simulink model "Flexible_Beam_LP_Modes_GenSS"  (R2017a)
settings: Solver=ode23t  StartTime=0.0  StopTime=200  RelTol=1e-3  AbsTol=1e-6  EnableMultiTasking=on
PreLoadFcn:
  | flexBeam_default_parameters
PostLoadFcn:
  | warning off Simulink:Engine:UsingDefaultMaxStepSize
  | warning off Simulink:Engine:SaveWithParameterizedLinks_Warning
undefined symbols (not defined in the file): beam_length, beam_wall, beam_width, Damping, density, Extr_Data_Box, extrusion_data_def, kbendingx, kbendingy, kelongz, ktwistz, num_elem, shearM, X, Y, youngsM, Z
libraries: sm_lib x307, nesl_utility x65
(part 1 of 9)
CloseFcn:
  | try,close(h1_Flexible_Beam_LP),end
  | clear h1_Flexible_Beam_LP
Description:
  | Lumped Parameter Beam for State Space Calculation
  | 
  | Copyright 2014-2017 The MathWorks, Inc.
settings Model: Creator=smiller  LastModifiedBy=smiller
settings DataIOCC: LimitDataPoints=on  SaveFormat=Array
settings OptimizationCC: LifeSpan=inf
settings DebuggingCC: UnderspecifiedInitializationDetection=Classic  MergeDetectMultiDrivingBlocksExec=none  SolverPrmCheckMsg=warning  AllowSymbolicDim=off  StateNameClashWarn=warning  SFUnexpectedBacktrackingDiag=warning  SFNoUnconditionalDefaultTransitionDiag=warning  SFExecutionAtInitializationDiag=none
settings HardwareCC: ProdBitPerPointer=32  ProdBitPerSizeT=32  ProdBitPerPtrDiffT=32  ProdLargestAtomicFloat=None  ProdIntDivRoundTo=Undefined  ProdEndianess=Unspecified  ProdWordSize=32  ProdHWDeviceType=32-bit Generic
settings ModelReferenceCC: PropagateSignalLabelsOutOfModel=off
settings GRTTargetCC: TargetLangStandard=C89/C90 (ANSI)  GeneratePreprocessorConditionals=Disable all
settings ConfigComp: CovMetricSettings=dw  CovHtmlReporting=on  CovSaveCumulativeToWorkspaceVar=on  CovSaveSingleToWorkspaceVar=on  CovExternalEMLEnable=off  CovSFcnEnable=off
settings ConfigurationSet: Description=SimMechanics 2G
settings ExplorerConfigSet: InternalSimMechanicsExplorerSettings="<ExplorerConfiguration><canonicalview>default</canonicalview><AnimationSetting><BasePlaybackSpeed>1.0</BasePlaybackSpeed><PlaybackSpeedFactor>1.0</PlaybackSpeedFactor></AnimationSetting><TilePanel><TileInfo><Tiles Columns=\"1\" Count=\"1\" Rows=\"1\"><Column Left=\"2\" Weight=\"1\"/><Column Left=\"626\"/><Row Top=\"2\" Weight=\"1\"/><Row Top=\"393\"/><Tile Height=\"1\" Width=\"1\" X=\"0\" Y=\"0\"/></Tiles></TileInfo><SceneInfo><SceneViewer><BGColor><R>0.60000002384185791</R><G>0.60000002384185791</G><B>0.60000002384185791</B></BGColor><Camera><Position><X>46.619711055341185</X><Y>-0.34983005837123721</Y><Z>0.38649668367083467</Z></Position><Center><X>15.061424751729401</X><Y>-0.47805428343950285</Y><Z>0.22325866927449958</Z></Center><Up><X>-0.0040752125209600008</X><Y>0.99998893056788307</Y><Z>0.0023518895830039648</Z></Up><Left>-1.9626362085342408</Left><Right>1.9626362085342408</Right><Bottom>-0.98671855330467229</Bottom><Top>0.98671855330467229</Top></Camera></SceneViewer></SceneInfo></TilePanel></ExplorerConfiguration>"

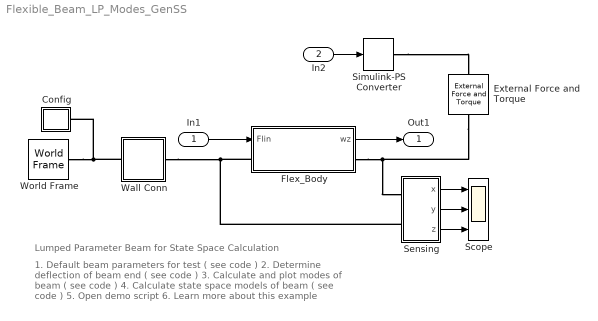
== system Flexible_Beam_LP_Modes_GenSS ==
  note: Lumped Parameter Beam for State Space Calculation
  note: 1. Default beam parameters for test ( see code )
      | 2. Determine deflection of beam end ( see code )
      | 3. Calculate and plot modes of beam ( see code )
      | 4. Calculate state space models of beam ( see code )
      | 5. Open demo script
      | 6. Learn more about this example
  In1 : Inport
  In2 : Inport  Port=2
  Config : Subsystem
  External Force and Torque : sm_lib/Forces and Torques/External Force and Torque  ForceResolutionFrame=AttachedFrame  EnableForceX=off  EnableForceY=on  EnableForceZ=off  EnableForce=off  TorqueResolutionFrame=AttachedFrame  EnableTorqueX=off  EnableTorqueY=off  EnableTorqueZ=off  EnableTorque=off
  Flex_Body : Subsystem  mask(Flexible Body){rho=density, youngsM=youngsM, shearM=shearM, b=Damping, popup_xc=Hollow Rectangle, beam_width=beam_width, beam_width_in=beam_width-2*beam_wall, beam_height=beam_width, beam_height_in=beam_width-2*beam_wall, circle_diameter=beam_width, circle_diameter_in=beam_width-2*beam_wall, custom_ixx=2.6121e-003, custom_iyy=2.6121e-003, custom_j=5.2242e-003, extrusion_data_custom=extrusion_data_def, beam_length=beam_length, numelem=num_elem, extrusion_data=Extr_Data_Box(beam_width,beam_width-2*beam_wall,beam_width,beam_width-2*beam_wall), radio_flextype=3-Axis Bending, Elongation, checkbox_lin=on}
      mask prompts: rho "Material Density (kg/(m^3)"; youngsM "Modulus of Elasticity (N/m2)"; shearM "Shear Modulus (N/m2)"; b "Damping Constant (Nm/rad.s)"; popup_xc "Cross-Section Type"; custom_ixx "Area Ixx"; custom_iyy "Area Iyy"; custom_j "Polar J"; extrusion_data_custom "Extrusion data [x;y] (m)"; beam_length "Length (m)"; numelem "Number of elements"; radio_flextype "Flexibility Type"; checkbox_lin "Add connections for linearization"
      mask help: Models a flexible beam based on lumped parameter method. Number of flexible elements, material properties as well as beam cross section and dimensions can be varied from mask parameters.
      mask init:
      | if(popup_xc==1)
      |     extrusion_data = Extr_Data_Box(beam_width,beam_width_in,beam_height,beam_height_in);
      |     xc_props = [beam_width beam_width_in beam_height beam_height_in];
      | elseif(popup_xc==2)
      |     extrusion_data = Extr_Data_Ring(circle_diameter/2,circle_diameter_in/2,0,360);
      |     xc_props = [circle_diameter circle_diameter_in];
      | elseif(popup_xc==3)
      |     extrusion_data = extrusion_data_custom;
      |     extrusion_data_vec = reshape(extrusion_data,[length(extrusion_data)*2,1]);
      |     xc_props = [custom_ixx;custom_iyy;custom_j;extrusion_data_vec];
      | end
      | 
      | [kbendingx, kbendingy, ktwistz, kelongz, length] = ...
      |     Compute_GFE_Prop(youngsM, shearM, numelem, beam_length,popup_xc,...
      |     xc_props);
      | 
      | flexBeam_lpar_construct_beam(gcb,numelem,radio_flextype,checkbox_lin);
      | 
      | state_order = flexBeam_lpar_getstateorder(gcb);
      | assignin('base','state_order',state_order);
      | 
      | clear xc_props
      settings: AttributesFormatString=No of Elem: 30  CopyFcn=set_param(gcb, 'LinkStatus', 'none')
      mask TypeOptions popup_xc: Hollow Rectangle | Hollow Circle | Custom
      mask Callback popup_xc:
      | maskObj = Simulink.Mask.get(gcb);
      | rcti_h = maskObj.getDialogControl('container_rectimage');
      | rctp_h = maskObj.getDialogControl('container_rectparams');
      | ciri_h = maskObj.getDialogControl('container_circleimage');
      | cirp_h = maskObj.getDialogControl('container_circleparams');
      | cusi_h = maskObj.getDialogControl('container_customimage');
      | cusp_h = maskObj.getDialogControl('container_customparams');
      | 
      | rcti_h.Visible = 'off';
      | rctp_h.Visible = 'off';
      | ciri_h.Visible = 'off';
      | cirp_h.Visible = 'off';
      | cusi_h.Visible = 'off';
      | cusp_h.Visible = 'off';
      | 
      | if strcmp(get_param(gcb,'popup_xc'),'Hollow Rectangle')
      |     rcti_h.Visible = 'on';
      |     rctp_h.Visible = 'on';
      | elseif strcmp(get_param(gcb,'popup_xc'),'Hollow Circle')
      |     ciri_h.Visible = 'on';
      |     cirp_h.Visible = 'on';
      | elseif strcmp(get_param(gcb,'popup_xc'),'Custom')
      |     cusi_h.Visible = 'on';
      |     cusp_h.Visible = 'on';
      | end
      | 
      | clear rcti_h rctp_h ciri_h cirp_h cusi_h cusp_h
      mask TypeOptions radio_flextype: 1-Axis Bending | 3-Axis Bending, Elongation
      mask DialogControl text_outer Prompt: Outer
      mask DialogControl text_inner Prompt: Inner
      mask DialogControl text_width Prompt: Width (m)
      mask DialogControl text_height Prompt: Height (m)
      mask DialogControl text_circle_outer Prompt: Outer
      mask DialogControl text_circle_inner Prompt: Inner
      mask DialogControl text_circle_width Prompt: Diameter (m)
      mask DialogControl text_moi Prompt: Moment of Inertia (m^4)
      mask DialogControl push_configBeam Prompt: Configure Beam
      mask DialogControl push_configBeam Callback:
      | thisblock = gcb;
      | v = get_param(thisblock,'MaskWSVariables');
      | getMaskValue = containers.Map({v.Name}',{v.Value}');
      | nelem = getMaskValue('numelem');
      | ftype = getMaskValue('radio_flextype');
      | flexBeam_lpar_construct_beam(thisblock,nelem,ftype,1)
      | %{
      | flexBeam_lpar_assemble_elements_4lin(thisblock,nelem);
      | ftype = getMaskValue('radio_flextype');
      | flexBeam_lpar_configure_flextype(thisblock,ftype);
      | %}
      | clear maskObj nel_h ftype thisblock
      mask Display: image(imread('Flexible_Beam.png'));
  Scope : Scope  NumInputPorts=3
  Sensing : Subsystem
  Simulink-PS Converter : nesl_utility/Simulink-PS Converter  PhysicalDomain=network_engine_domain  SubClassName=ps_input  LeftPortType=input  RightPortType=output  PseudoPeriodic=off  Frequencies=[]  NoiseDistribution=none  NoiseParameters=[]  Unit=1  AffineConversion=off  FilteringAndDerivatives=zero  SimscapeFilterOrder=1  InputFilterTimeConstant=0.001  UdotUserProvided=1
  Wall Conn : Subsystem  Variant=on  OverrideUsingVariant=Rotate
      mask Display:
      | blk = find_system(gcbh, 'SearchDepth', 1, 'Parent', gcb, 'VariantObject', get_param(gcb,'activevariant'));
      | eval(get_param(blk, 'MaskDisplay'));
  World Frame : sm_lib/Frames and Transforms/World Frame
  Out1 : Outport
  wires:
  In2/1 -> Simulink-PS Converter/1
  Sensing/1(x) -> Scope/1
  Sensing/2(y) -> Scope/2
  Sensing/3(z) -> Scope/3
  In1/1 -> Flex_Body/1(Flin)
  Flex_Body/1(wz) -> Out1/1
  connections:
  Simulink-PS Converter/RConn1 -- External Force and Torque/LConn1
  External Force and Torque/RConn1 -- Flex_Body/RConn1 -- Sensing/LConn1
  Sensing/LConn2 -- Flex_Body/LConn1 -- Wall Conn/RConn1
  World Frame/RConn1 -- Config/LConn1 -- Wall Conn/LConn1

== system Flexible_Beam_LP_Modes_GenSS/Config ==
  Mechanism Configuration : sm_lib/Utilities/Mechanism Configuration  UniformGravity=Constant  GravityVector=gravity  GravityUnits=m/s^2  LinearizationDelta=0.001
  Solver Configuration : nesl_utility/Solver Configuration  PhysicalDomain=network_engine_domain  SubClassName=solver  LeftPortType=input  RightPortType=generic  Accelerate=off  Tones=[]  Harmonics=[]  SimulateNoise=off  Profile=off  UseLocalSampling=off  EnableSwitchedLinearOptims=on  FrequencyDomain=off  UseCCode=off  RelTol=0.001  AbsTol=1e-06  MinStep=1e-09  ToWorkspace=off  RevertToSquareIcSolve=off  NumHomotopyIterations=100  PhasorMode=off  PhasorModeNumHarmonics=1  OverrideAbsTol=off  DoDC=off  ResidualTolerance=1e-09  UseLocalSolver=off  LocalSolverChoice=NE_BACKWARD_EULER_ADVANCER  LocalSolverSampleTime=0.001  DoFixedCost=off  MaxNonlinIter=3  MaxModeIter=2  LinearAlgebra=Sparse  DelaysMemoryBudget=1024  AutomaticFiltering=on  FilteringTimeConstant=0.001
  C : PMIOPort  Port=1  Side=Left
  connections:
  Mechanism Configuration/RConn1 -- Solver Configuration/RConn1 -- C/RConn1

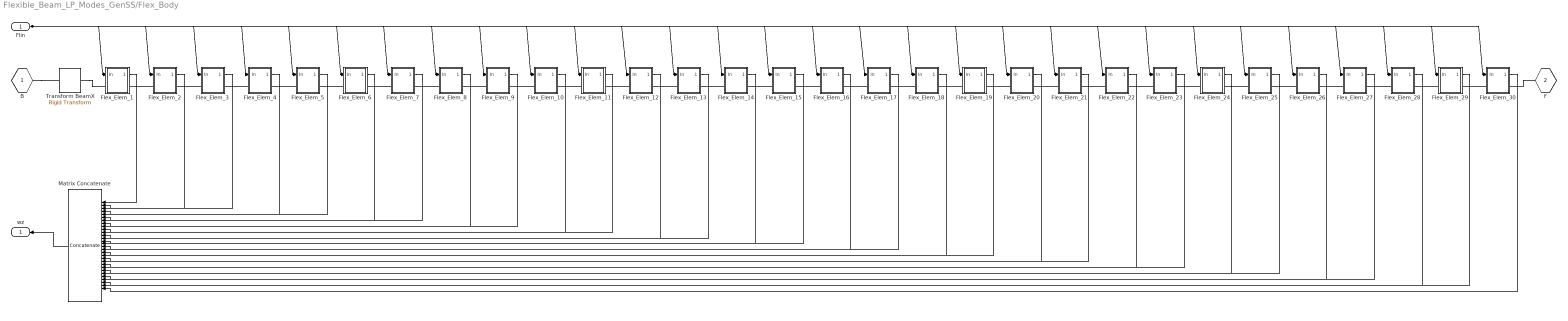
== system Flexible_Beam_LP_Modes_GenSS/Flex_Body ==
  Flin : Inport
  Flex_Elem_1 : Subsystem  VariantControl=Bend  mask{length=length, rho=rho, beam_width=beam_width, beam_wall=beam_wall, kbendingx=kbendingx, kbendingy=kbendingy, kbendingz=ktwistz, kelongz=kelongz, b=b}
      mask prompts: length "Beam Length (m)"; rho "Material Density (kg/(m^3)"; beam_width "Beam Width & Height (m)"; beam_wall "Beam Wall Thickness (m)"; kbendingx "Bending Spring Constant about X(Nm/rad)"; kbendingy "Bending Spring Constant about Y(Nm/rad)"; kbendingz "Twist Spring Constant about Z(Nm/rad)"; kelongz "Elongation Spring Constant about Z(N/m)"; b "Damping Constant (Nm/rad.s)"
      settings: CopyFcn=set_param(gcb, 'LinkStatus', 'none')
  Flex_Elem_10 : Subsystem  VariantControl=Bend  mask{length=length, rho=rho, beam_width=beam_width, beam_wall=beam_wall, kbendingx=kbendingx, kbendingy=kbendingy, kbendingz=ktwistz, kelongz=kelongz, b=b}
      mask prompts: length "Beam Length (m)"; rho "Material Density (kg/(m^3)"; beam_width "Beam Width & Height (m)"; beam_wall "Beam Wall Thickness (m)"; kbendingx "Bending Spring Constant about X(Nm/rad)"; kbendingy "Bending Spring Constant about Y(Nm/rad)"; kbendingz "Twist Spring Constant about Z(Nm/rad)"; kelongz "Elongation Spring Constant about Z(N/m)"; b "Damping Constant (Nm/rad.s)"
      settings: CopyFcn=set_param(gcb, 'LinkStatus', 'none')
  Flex_Elem_11 : Subsystem  VariantControl=Bend  mask{length=length, rho=rho, beam_width=beam_width, beam_wall=beam_wall, kbendingx=kbendingx, kbendingy=kbendingy, kbendingz=ktwistz, kelongz=kelongz, b=b}
      mask prompts: length "Beam Length (m)"; rho "Material Density (kg/(m^3)"; beam_width "Beam Width & Height (m)"; beam_wall "Beam Wall Thickness (m)"; kbendingx "Bending Spring Constant about X(Nm/rad)"; kbendingy "Bending Spring Constant about Y(Nm/rad)"; kbendingz "Twist Spring Constant about Z(Nm/rad)"; kelongz "Elongation Spring Constant about Z(N/m)"; b "Damping Constant (Nm/rad.s)"
      settings: CopyFcn=set_param(gcb, 'LinkStatus', 'none')
  Flex_Elem_12 : Subsystem  VariantControl=Bend  mask{length=length, rho=rho, beam_width=beam_width, beam_wall=beam_wall, kbendingx=kbendingx, kbendingy=kbendingy, kbendingz=ktwistz, kelongz=kelongz, b=b}
      mask prompts: length "Beam Length (m)"; rho "Material Density (kg/(m^3)"; beam_width "Beam Width & Height (m)"; beam_wall "Beam Wall Thickness (m)"; kbendingx "Bending Spring Constant about X(Nm/rad)"; kbendingy "Bending Spring Constant about Y(Nm/rad)"; kbendingz "Twist Spring Constant about Z(Nm/rad)"; kelongz "Elongation Spring Constant about Z(N/m)"; b "Damping Constant (Nm/rad.s)"
      settings: CopyFcn=set_param(gcb, 'LinkStatus', 'none')
  Flex_Elem_13 : Subsystem  VariantControl=Bend  mask{length=length, rho=rho, beam_width=beam_width, beam_wall=beam_wall, kbendingx=kbendingx, kbendingy=kbendingy, kbendingz=ktwistz, kelongz=kelongz, b=b}
      mask prompts: length "Beam Length (m)"; rho "Material Density (kg/(m^3)"; beam_width "Beam Width & Height (m)"; beam_wall "Beam Wall Thickness (m)"; kbendingx "Bending Spring Constant about X(Nm/rad)"; kbendingy "Bending Spring Constant about Y(Nm/rad)"; kbendingz "Twist Spring Constant about Z(Nm/rad)"; kelongz "Elongation Spring Constant about Z(N/m)"; b "Damping Constant (Nm/rad.s)"
      settings: CopyFcn=set_param(gcb, 'LinkStatus', 'none')
  Flex_Elem_14 : Subsystem  VariantControl=Bend  mask{length=length, rho=rho, beam_width=beam_width, beam_wall=beam_wall, kbendingx=kbendingx, kbendingy=kbendingy, kbendingz=ktwistz, kelongz=kelongz, b=b}
      mask prompts: length "Beam Length (m)"; rho "Material Density (kg/(m^3)"; beam_width "Beam Width & Height (m)"; beam_wall "Beam Wall Thickness (m)"; kbendingx "Bending Spring Constant about X(Nm/rad)"; kbendingy "Bending Spring Constant about Y(Nm/rad)"; kbendingz "Twist Spring Constant about Z(Nm/rad)"; kelongz "Elongation Spring Constant about Z(N/m)"; b "Damping Constant (Nm/rad.s)"
      settings: CopyFcn=set_param(gcb, 'LinkStatus', 'none')
  Flex_Elem_15 : Subsystem  VariantControl=Bend  mask{length=length, rho=rho, beam_width=beam_width, beam_wall=beam_wall, kbendingx=kbendingx, kbendingy=kbendingy, kbendingz=ktwistz, kelongz=kelongz, b=b}
      mask prompts: length "Beam Length (m)"; rho "Material Density (kg/(m^3)"; beam_width "Beam Width & Height (m)"; beam_wall "Beam Wall Thickness (m)"; kbendingx "Bending Spring Constant about X(Nm/rad)"; kbendingy "Bending Spring Constant about Y(Nm/rad)"; kbendingz "Twist Spring Constant about Z(Nm/rad)"; kelongz "Elongation Spring Constant about Z(N/m)"; b "Damping Constant (Nm/rad.s)"
      settings: CopyFcn=set_param(gcb, 'LinkStatus', 'none')
  Flex_Elem_16 : Subsystem  VariantControl=Bend  mask{length=length, rho=rho, beam_width=beam_width, beam_wall=beam_wall, kbendingx=kbendingx, kbendingy=kbendingy, kbendingz=ktwistz, kelongz=kelongz, b=b}
      mask prompts: length "Beam Length (m)"; rho "Material Density (kg/(m^3)"; beam_width "Beam Width & Height (m)"; beam_wall "Beam Wall Thickness (m)"; kbendingx "Bending Spring Constant about X(Nm/rad)"; kbendingy "Bending Spring Constant about Y(Nm/rad)"; kbendingz "Twist Spring Constant about Z(Nm/rad)"; kelongz "Elongation Spring Constant about Z(N/m)"; b "Damping Constant (Nm/rad.s)"
      settings: CopyFcn=set_param(gcb, 'LinkStatus', 'none')
  Flex_Elem_17 : Subsystem  VariantControl=Bend  mask{length=length, rho=rho, beam_width=beam_width, beam_wall=beam_wall, kbendingx=kbendingx, kbendingy=kbendingy, kbendingz=ktwistz, kelongz=kelongz, b=b}
      mask prompts: length "Beam Length (m)"; rho "Material Density (kg/(m^3)"; beam_width "Beam Width & Height (m)"; beam_wall "Beam Wall Thickness (m)"; kbendingx "Bending Spring Constant about X(Nm/rad)"; kbendingy "Bending Spring Constant about Y(Nm/rad)"; kbendingz "Twist Spring Constant about Z(Nm/rad)"; kelongz "Elongation Spring Constant about Z(N/m)"; b "Damping Constant (Nm/rad.s)"
      settings: CopyFcn=set_param(gcb, 'LinkStatus', 'none')
  Flex_Elem_18 : Subsystem  VariantControl=Bend  mask{length=length, rho=rho, beam_width=beam_width, beam_wall=beam_wall, kbendingx=kbendingx, kbendingy=kbendingy, kbendingz=ktwistz, kelongz=kelongz, b=b}
      mask prompts: length "Beam Length (m)"; rho "Material Density (kg/(m^3)"; beam_width "Beam Width & Height (m)"; beam_wall "Beam Wall Thickness (m)"; kbendingx "Bending Spring Constant about X(Nm/rad)"; kbendingy "Bending Spring Constant about Y(Nm/rad)"; kbendingz "Twist Spring Constant about Z(Nm/rad)"; kelongz "Elongation Spring Constant about Z(N/m)"; b "Damping Constant (Nm/rad.s)"
      settings: CopyFcn=set_param(gcb, 'LinkStatus', 'none')
  Flex_Elem_19 : Subsystem  VariantControl=Bend  mask{length=length, rho=rho, beam_width=beam_width, beam_wall=beam_wall, kbendingx=kbendingx, kbendingy=kbendingy, kbendingz=ktwistz, kelongz=kelongz, b=b}
      mask prompts: length "Beam Length (m)"; rho "Material Density (kg/(m^3)"; beam_width "Beam Width & Height (m)"; beam_wall "Beam Wall Thickness (m)"; kbendingx "Bending Spring Constant about X(Nm/rad)"; kbendingy "Bending Spring Constant about Y(Nm/rad)"; kbendingz "Twist Spring Constant about Z(Nm/rad)"; kelongz "Elongation Spring Constant about Z(N/m)"; b "Damping Constant (Nm/rad.s)"
      settings: CopyFcn=set_param(gcb, 'LinkStatus', 'none')
  Flex_Elem_2 : Subsystem  VariantControl=Bend  mask{length=length, rho=rho, beam_width=beam_width, beam_wall=beam_wall, kbendingx=kbendingx, kbendingy=kbendingy, kbendingz=ktwistz, kelongz=kelongz, b=b}
      mask prompts: length "Beam Length (m)"; rho "Material Density (kg/(m^3)"; beam_width "Beam Width & Height (m)"; beam_wall "Beam Wall Thickness (m)"; kbendingx "Bending Spring Constant about X(Nm/rad)"; kbendingy "Bending Spring Constant about Y(Nm/rad)"; kbendingz "Twist Spring Constant about Z(Nm/rad)"; kelongz "Elongation Spring Constant about Z(N/m)"; b "Damping Constant (Nm/rad.s)"
      settings: CopyFcn=set_param(gcb, 'LinkStatus', 'none')
  Flex_Elem_20 : Subsystem  VariantControl=Bend  mask{length=length, rho=rho, beam_width=beam_width, beam_wall=beam_wall, kbendingx=kbendingx, kbendingy=kbendingy, kbendingz=ktwistz, kelongz=kelongz, b=b}
      mask prompts: length "Beam Length (m)"; rho "Material Density (kg/(m^3)"; beam_width "Beam Width & Height (m)"; beam_wall "Beam Wall Thickness (m)"; kbendingx "Bending Spring Constant about X(Nm/rad)"; kbendingy "Bending Spring Constant about Y(Nm/rad)"; kbendingz "Twist Spring Constant about Z(Nm/rad)"; kelongz "Elongation Spring Constant about Z(N/m)"; b "Damping Constant (Nm/rad.s)"
      settings: CopyFcn=set_param(gcb, 'LinkStatus', 'none')
  Flex_Elem_21 : Subsystem  VariantControl=Bend  mask{length=length, rho=rho, beam_width=beam_width, beam_wall=beam_wall, kbendingx=kbendingx, kbendingy=kbendingy, kbendingz=ktwistz, kelongz=kelongz, b=b}
      mask prompts: length "Beam Length (m)"; rho "Material Density (kg/(m^3)"; beam_width "Beam Width & Height (m)"; beam_wall "Beam Wall Thickness (m)"; kbendingx "Bending Spring Constant about X(Nm/rad)"; kbendingy "Bending Spring Constant about Y(Nm/rad)"; kbendingz "Twist Spring Constant about Z(Nm/rad)"; kelongz "Elongation Spring Constant about Z(N/m)"; b "Damping Constant (Nm/rad.s)"
      settings: CopyFcn=set_param(gcb, 'LinkStatus', 'none')
  Flex_Elem_22 : Subsystem  VariantControl=Bend  mask{length=length, rho=rho, beam_width=beam_width, beam_wall=beam_wall, kbendingx=kbendingx, kbendingy=kbendingy, kbendingz=ktwistz, kelongz=kelongz, b=b}
      mask prompts: length "Beam Length (m)"; rho "Material Density (kg/(m^3)"; beam_width "Beam Width & Height (m)"; beam_wall "Beam Wall Thickness (m)"; kbendingx "Bending Spring Constant about X(Nm/rad)"; kbendingy "Bending Spring Constant about Y(Nm/rad)"; kbendingz "Twist Spring Constant about Z(Nm/rad)"; kelongz "Elongation Spring Constant about Z(N/m)"; b "Damping Constant (Nm/rad.s)"
      settings: CopyFcn=set_param(gcb, 'LinkStatus', 'none')
  Flex_Elem_23 : Subsystem  VariantControl=Bend  mask{length=length, rho=rho, beam_width=beam_width, beam_wall=beam_wall, kbendingx=kbendingx, kbendingy=kbendingy, kbendingz=ktwistz, kelongz=kelongz, b=b}
      mask prompts: length "Beam Length (m)"; rho "Material Density (kg/(m^3)"; beam_width "Beam Width & Height (m)"; beam_wall "Beam Wall Thickness (m)"; kbendingx "Bending Spring Constant about X(Nm/rad)"; kbendingy "Bending Spring Constant about Y(Nm/rad)"; kbendingz "Twist Spring Constant about Z(Nm/rad)"; kelongz "Elongation Spring Constant about Z(N/m)"; b "Damping Constant (Nm/rad.s)"
      settings: CopyFcn=set_param(gcb, 'LinkStatus', 'none')
  Flex_Elem_24 : Subsystem  VariantControl=Bend  mask{length=length, rho=rho, beam_width=beam_width, beam_wall=beam_wall, kbendingx=kbendingx, kbendingy=kbendingy, kbendingz=ktwistz, kelongz=kelongz, b=b}
      mask prompts: length "Beam Length (m)"; rho "Material Density (kg/(m^3)"; beam_width "Beam Width & Height (m)"; beam_wall "Beam Wall Thickness (m)"; kbendingx "Bending Spring Constant about X(Nm/rad)"; kbendingy "Bending Spring Constant about Y(Nm/rad)"; kbendingz "Twist Spring Constant about Z(Nm/rad)"; kelongz "Elongation Spring Constant about Z(N/m)"; b "Damping Constant (Nm/rad.s)"
      settings: CopyFcn=set_param(gcb, 'LinkStatus', 'none')
  Flex_Elem_25 : Subsystem  VariantControl=Bend  mask{length=length, rho=rho, beam_width=beam_width, beam_wall=beam_wall, kbendingx=kbendingx, kbendingy=kbendingy, kbendingz=ktwistz, kelongz=kelongz, b=b}
      mask prompts: length "Beam Length (m)"; rho "Material Density (kg/(m^3)"; beam_width "Beam Width & Height (m)"; beam_wall "Beam Wall Thickness (m)"; kbendingx "Bending Spring Constant about X(Nm/rad)"; kbendingy "Bending Spring Constant about Y(Nm/rad)"; kbendingz "Twist Spring Constant about Z(Nm/rad)"; kelongz "Elongation Spring Constant about Z(N/m)"; b "Damping Constant (Nm/rad.s)"
      settings: CopyFcn=set_param(gcb, 'LinkStatus', 'none')
  Flex_Elem_26 : Subsystem  VariantControl=Bend  mask{length=length, rho=rho, beam_width=beam_width, beam_wall=beam_wall, kbendingx=kbendingx, kbendingy=kbendingy, kbendingz=ktwistz, kelongz=kelongz, b=b}
      mask prompts: length "Beam Length (m)"; rho "Material Density (kg/(m^3)"; beam_width "Beam Width & Height (m)"; beam_wall "Beam Wall Thickness (m)"; kbendingx "Bending Spring Constant about X(Nm/rad)"; kbendingy "Bending Spring Constant about Y(Nm/rad)"; kbendingz "Twist Spring Constant about Z(Nm/rad)"; kelongz "Elongation Spring Constant about Z(N/m)"; b "Damping Constant (Nm/rad.s)"
      settings: CopyFcn=set_param(gcb, 'LinkStatus', 'none')
  Flex_Elem_27 : Subsystem  VariantControl=Bend  mask{length=length, rho=rho, beam_width=beam_width, beam_wall=beam_wall, kbendingx=kbendingx, kbendingy=kbendingy, kbendingz=ktwistz, kelongz=kelongz, b=b}
      mask prompts: length "Beam Length (m)"; rho "Material Density (kg/(m^3)"; beam_width "Beam Width & Height (m)"; beam_wall "Beam Wall Thickness (m)"; kbendingx "Bending Spring Constant about X(Nm/rad)"; kbendingy "Bending Spring Constant about Y(Nm/rad)"; kbendingz "Twist Spring Constant about Z(Nm/rad)"; kelongz "Elongation Spring Constant about Z(N/m)"; b "Damping Constant (Nm/rad.s)"
      settings: CopyFcn=set_param(gcb, 'LinkStatus', 'none')
  Flex_Elem_28 : Subsystem  VariantControl=Bend  mask{length=length, rho=rho, beam_width=beam_width, beam_wall=beam_wall, kbendingx=kbendingx, kbendingy=kbendingy, kbendingz=ktwistz, kelongz=kelongz, b=b}
      mask prompts: length "Beam Length (m)"; rho "Material Density (kg/(m^3)"; beam_width "Beam Width & Height (m)"; beam_wall "Beam Wall Thickness (m)"; kbendingx "Bending Spring Constant about X(Nm/rad)"; kbendingy "Bending Spring Constant about Y(Nm/rad)"; kbendingz "Twist Spring Constant about Z(Nm/rad)"; kelongz "Elongation Spring Constant about Z(N/m)"; b "Damping Constant (Nm/rad.s)"
      settings: CopyFcn=set_param(gcb, 'LinkStatus', 'none')
  Flex_Elem_29 : Subsystem  VariantControl=Bend  mask{length=length, rho=rho, beam_width=beam_width, beam_wall=beam_wall, kbendingx=kbendingx, kbendingy=kbendingy, kbendingz=ktwistz, kelongz=kelongz, b=b}
      mask prompts: length "Beam Length (m)"; rho "Material Density (kg/(m^3)"; beam_width "Beam Width & Height (m)"; beam_wall "Beam Wall Thickness (m)"; kbendingx "Bending Spring Constant about X(Nm/rad)"; kbendingy "Bending Spring Constant about Y(Nm/rad)"; kbendingz "Twist Spring Constant about Z(Nm/rad)"; kelongz "Elongation Spring Constant about Z(N/m)"; b "Damping Constant (Nm/rad.s)"
      settings: CopyFcn=set_param(gcb, 'LinkStatus', 'none')
  Flex_Elem_3 : Subsystem  VariantControl=Bend  mask{length=length, rho=rho, beam_width=beam_width, beam_wall=beam_wall, kbendingx=kbendingx, kbendingy=kbendingy, kbendingz=ktwistz, kelongz=kelongz, b=b}
      mask prompts: length "Beam Length (m)"; rho "Material Density (kg/(m^3)"; beam_width "Beam Width & Height (m)"; beam_wall "Beam Wall Thickness (m)"; kbendingx "Bending Spring Constant about X(Nm/rad)"; kbendingy "Bending Spring Constant about Y(Nm/rad)"; kbendingz "Twist Spring Constant about Z(Nm/rad)"; kelongz "Elongation Spring Constant about Z(N/m)"; b "Damping Constant (Nm/rad.s)"
      settings: CopyFcn=set_param(gcb, 'LinkStatus', 'none')
  Flex_Elem_30 : Subsystem  VariantControl=Bend  mask{length=length, rho=rho, beam_width=beam_width, beam_wall=beam_wall, kbendingx=kbendingx, kbendingy=kbendingy, kbendingz=ktwistz, kelongz=kelongz, b=b}
      mask prompts: length "Beam Length (m)"; rho "Material Density (kg/(m^3)"; beam_width "Beam Width & Height (m)"; beam_wall "Beam Wall Thickness (m)"; kbendingx "Bending Spring Constant about X(Nm/rad)"; kbendingy "Bending Spring Constant about Y(Nm/rad)"; kbendingz "Twist Spring Constant about Z(Nm/rad)"; kelongz "Elongation Spring Constant about Z(N/m)"; b "Damping Constant (Nm/rad.s)"
      settings: CopyFcn=set_param(gcb, 'LinkStatus', 'none')
  Flex_Elem_4 : Subsystem  VariantControl=Bend  mask{length=length, rho=rho, beam_width=beam_width, beam_wall=beam_wall, kbendingx=kbendingx, kbendingy=kbendingy, kbendingz=ktwistz, kelongz=kelongz, b=b}
      mask prompts: length "Beam Length (m)"; rho "Material Density (kg/(m^3)"; beam_width "Beam Width & Height (m)"; beam_wall "Beam Wall Thickness (m)"; kbendingx "Bending Spring Constant about X(Nm/rad)"; kbendingy "Bending Spring Constant about Y(Nm/rad)"; kbendingz "Twist Spring Constant about Z(Nm/rad)"; kelongz "Elongation Spring Constant about Z(N/m)"; b "Damping Constant (Nm/rad.s)"
      settings: CopyFcn=set_param(gcb, 'LinkStatus', 'none')
  Flex_Elem_5 : Subsystem  VariantControl=Bend  mask{length=length, rho=rho, beam_width=beam_width, beam_wall=beam_wall, kbendingx=kbendingx, kbendingy=kbendingy, kbendingz=ktwistz, kelongz=kelongz, b=b}
      mask prompts: length "Beam Length (m)"; rho "Material Density (kg/(m^3)"; beam_width "Beam Width & Height (m)"; beam_wall "Beam Wall Thickness (m)"; kbendingx "Bending Spring Constant about X(Nm/rad)"; kbendingy "Bending Spring Constant about Y(Nm/rad)"; kbendingz "Twist Spring Constant about Z(Nm/rad)"; kelongz "Elongation Spring Constant about Z(N/m)"; b "Damping Constant (Nm/rad.s)"
      settings: CopyFcn=set_param(gcb, 'LinkStatus', 'none')
  Flex_Elem_6 : Subsystem  VariantControl=Bend  mask{length=length, rho=rho, beam_width=beam_width, beam_wall=beam_wall, kbendingx=kbendingx, kbendingy=kbendingy, kbendingz=ktwistz, kelongz=kelongz, b=b}
      mask prompts: length "Beam Length (m)"; rho "Material Density (kg/(m^3)"; beam_width "Beam Width & Height (m)"; beam_wall "Beam Wall Thickness (m)"; kbendingx "Bending Spring Constant about X(Nm/rad)"; kbendingy "Bending Spring Constant about Y(Nm/rad)"; kbendingz "Twist Spring Constant about Z(Nm/rad)"; kelongz "Elongation Spring Constant about Z(N/m)"; b "Damping Constant (Nm/rad.s)"
      settings: CopyFcn=set_param(gcb, 'LinkStatus', 'none')
  Flex_Elem_7 : Subsystem  VariantControl=Bend  mask{length=length, rho=rho, beam_width=beam_width, beam_wall=beam_wall, kbendingx=kbendingx, kbendingy=kbendingy, kbendingz=ktwistz, kelongz=kelongz, b=b}
      mask prompts: length "Beam Length (m)"; rho "Material Density (kg/(m^3)"; beam_width "Beam Width & Height (m)"; beam_wall "Beam Wall Thickness (m)"; kbendingx "Bending Spring Constant about X(Nm/rad)"; kbendingy "Bending Spring Constant about Y(Nm/rad)"; kbendingz "Twist Spring Constant about Z(Nm/rad)"; kelongz "Elongation Spring Constant about Z(N/m)"; b "Damping Constant (Nm/rad.s)"
      settings: CopyFcn=set_param(gcb, 'LinkStatus', 'none')
  Flex_Elem_8 : Subsystem  VariantControl=Bend  mask{length=length, rho=rho, beam_width=beam_width, beam_wall=beam_wall, kbendingx=kbendingx, kbendingy=kbendingy, kbendingz=ktwistz, kelongz=kelongz, b=b}
      mask prompts: length "Beam Length (m)"; rho "Material Density (kg/(m^3)"; beam_width "Beam Width & Height (m)"; beam_wall "Beam Wall Thickness (m)"; kbendingx "Bending Spring Constant about X(Nm/rad)"; kbendingy "Bending Spring Constant about Y(Nm/rad)"; kbendingz "Twist Spring Constant about Z(Nm/rad)"; kelongz "Elongation Spring Constant about Z(N/m)"; b "Damping Constant (Nm/rad.s)"
      settings: CopyFcn=set_param(gcb, 'LinkStatus', 'none')
  Flex_Elem_9 : Subsystem  VariantControl=Bend  mask{length=length, rho=rho, beam_width=beam_width, beam_wall=beam_wall, kbendingx=kbendingx, kbendingy=kbendingy, kbendingz=ktwistz, kelongz=kelongz, b=b}
      mask prompts: length "Beam Length (m)"; rho "Material Density (kg/(m^3)"; beam_width "Beam Width & Height (m)"; beam_wall "Beam Wall Thickness (m)"; kbendingx "Bending Spring Constant about X(Nm/rad)"; kbendingy "Bending Spring Constant about Y(Nm/rad)"; kbendingz "Twist Spring Constant about Z(Nm/rad)"; kelongz "Elongation Spring Constant about Z(N/m)"; b "Damping Constant (Nm/rad.s)"
      settings: CopyFcn=set_param(gcb, 'LinkStatus', 'none')
  Matrix Concatenate : Concatenate  NumInputs=numelem  Mode=Multidimensional array
  Transform BeamX : sm_lib/Frames and Transforms/Rigid Transform  TranslationMethod=StandardAxis  TranslationStandardOffset=0  TranslationLengthUnit=m  TranslationStandardAxis=+Z  TranslationCartesianOffset=[0 0 0]  TranslationROffset=0  TranslationROffsetUnits=m  TranslationZOffset=0  TranslationZOffsetUnits=m  TranslationThetaOffset=0  TranslationThetaOffsetUnits=deg  RotationMethod=StandardAxis  RotationAngleUnits=deg  RotationStandardAxis=+Y  RotationAngle=90  RotationArbitraryAxis=[0 0 1]  FollAlignAxisA=+X  BaseAlignAxisA=+Y  FollAlignAxisB=+Y  BaseAlignAxisB=+Z  RotationSequenceAxes=FollowerAxes  RotationSequence=XYX  RotationSequenceAngles=[0 0 0]  RotationSequenceAnglesUnits=deg  RotationMatrix=[1 0 0; 0 1 0; 0 0 1]
  B : PMIOPort  Port=1  Side=Left
  F : PMIOPort  Port=2  Side=Right
  wz : Outport
  wires:
  Flin/1 -> Flex_Elem_1/1(In), Flex_Elem_2/1(In), Flex_Elem_3/1(In), Flex_Elem_4/1(In), Flex_Elem_5/1(In), Flex_Elem_6/1(In), Flex_Elem_7/1(In), Flex_Elem_8/1(In), Flex_Elem_9/1(In), Flex_Elem_10/1(In), Flex_Elem_11/1(In), Flex_Elem_12/1(In), Flex_Elem_13/1(In), Flex_Elem_14/1(In), Flex_Elem_15/1(In), Flex_Elem_16/1(In), Flex_Elem_17/1(In), Flex_Elem_18/1(In), Flex_Elem_19/1(In), Flex_Elem_20/1(In), Flex_Elem_21/1(In), Flex_Elem_22/1(In), Flex_Elem_23/1(In), Flex_Elem_24/1(In), Flex_Elem_25/1(In), Flex_Elem_26/1(In), Flex_Elem_27/1(In), Flex_Elem_28/1(In), Flex_Elem_29/1(In), Flex_Elem_30/1(In)
  Flex_Elem_1/1(Out) -> Matrix Concatenate/1
  Flex_Elem_2/1(Out) -> Matrix Concatenate/2
  Flex_Elem_3/1(Out) -> Matrix Concatenate/3
  Flex_Elem_4/1(Out) -> Matrix Concatenate/4
  Flex_Elem_5/1(Out) -> Matrix Concatenate/5
  Flex_Elem_6/1(Out) -> Matrix Concatenate/6
  Flex_Elem_7/1(Out) -> Matrix Concatenate/7
  Flex_Elem_8/1(Out) -> Matrix Concatenate/8
  Flex_Elem_9/1(Out) -> Matrix Concatenate/9
  Flex_Elem_10/1(Out) -> Matrix Concatenate/10
  Flex_Elem_11/1(Out) -> Matrix Concatenate/11
  Flex_Elem_12/1(Out) -> Matrix Concatenate/12
  Flex_Elem_13/1(Out) -> Matrix Concatenate/13
  Flex_Elem_14/1(Out) -> Matrix Concatenate/14
  Flex_Elem_15/1(Out) -> Matrix Concatenate/15
  Flex_Elem_16/1(Out) -> Matrix Concatenate/16
  Flex_Elem_17/1(Out) -> Matrix Concatenate/17
  Flex_Elem_18/1(Out) -> Matrix Concatenate/18
  Flex_Elem_19/1(Out) -> Matrix Concatenate/19
  Flex_Elem_20/1(Out) -> Matrix Concatenate/20
  Flex_Elem_21/1(Out) -> Matrix Concatenate/21
  Flex_Elem_22/1(Out) -> Matrix Concatenate/22
  Flex_Elem_23/1(Out) -> Matrix Concatenate/23
  Flex_Elem_24/1(Out) -> Matrix Concatenate/24
  Flex_Elem_25/1(Out) -> Matrix Concatenate/25
  Flex_Elem_26/1(Out) -> Matrix Concatenate/26
  Flex_Elem_27/1(Out) -> Matrix Concatenate/27
  Flex_Elem_28/1(Out) -> Matrix Concatenate/28
  Flex_Elem_29/1(Out) -> Matrix Concatenate/29
  Flex_Elem_30/1(Out) -> Matrix Concatenate/30
  Matrix Concatenate/1 -> wz/1
  connections:
  B/RConn1 -- Transform BeamX/LConn1
  Transform BeamX/RConn1 -- Flex_Elem_1/LConn1
  Flex_Elem_1/RConn1 -- Flex_Elem_2/LConn1
  Flex_Elem_2/RConn1 -- Flex_Elem_3/LConn1
  Flex_Elem_3/RConn1 -- Flex_Elem_4/LConn1
  Flex_Elem_4/RConn1 -- Flex_Elem_5/LConn1
  Flex_Elem_5/RConn1 -- Flex_Elem_6/LConn1
  Flex_Elem_6/RConn1 -- Flex_Elem_7/LConn1
  Flex_Elem_7/RConn1 -- Flex_Elem_8/LConn1
  Flex_Elem_8/RConn1 -- Flex_Elem_9/LConn1
  Flex_Elem_9/RConn1 -- Flex_Elem_10/LConn1
  Flex_Elem_10/RConn1 -- Flex_Elem_11/LConn1
  Flex_Elem_11/RConn1 -- Flex_Elem_12/LConn1
  Flex_Elem_12/RConn1 -- Flex_Elem_13/LConn1
  Flex_Elem_13/RConn1 -- Flex_Elem_14/LConn1
  Flex_Elem_14/RConn1 -- Flex_Elem_15/LConn1
  Flex_Elem_15/RConn1 -- Flex_Elem_16/LConn1
  Flex_Elem_16/RConn1 -- Flex_Elem_17/LConn1
  Flex_Elem_17/RConn1 -- Flex_Elem_18/LConn1
  Flex_Elem_18/RConn1 -- Flex_Elem_19/LConn1
  Flex_Elem_19/RConn1 -- Flex_Elem_20/LConn1
  Flex_Elem_20/RConn1 -- Flex_Elem_21/LConn1
  Flex_Elem_21/RConn1 -- Flex_Elem_22/LConn1
  Flex_Elem_22/RConn1 -- Flex_Elem_23/LConn1
  Flex_Elem_23/RConn1 -- Flex_Elem_24/LConn1
  Flex_Elem_24/RConn1 -- Flex_Elem_25/LConn1
  Flex_Elem_25/RConn1 -- Flex_Elem_26/LConn1
  Flex_Elem_26/RConn1 -- Flex_Elem_27/LConn1
  Flex_Elem_27/RConn1 -- Flex_Elem_28/LConn1
  Flex_Elem_28/RConn1 -- Flex_Elem_29/LConn1
  Flex_Elem_29/RConn1 -- Flex_Elem_30/LConn1
  Flex_Elem_30/RConn1 -- F/RConn1

== system Flexible_Beam_LP_Modes_GenSS/Sensing ==
  PS-Simulink Converter : nesl_utility/PS-Simulink Converter  PhysicalDomain=network_engine_domain  SubClassName=ps_output  LeftPortType=input  RightPortType=output  PseudoPeriodic=off  Frequencies=[]  Unit=1  AffineConversion=off
  PS-Simulink Converter1 : nesl_utility/PS-Simulink Converter  PhysicalDomain=network_engine_domain  SubClassName=ps_output  LeftPortType=input  RightPortType=output  PseudoPeriodic=off  Frequencies=[]  Unit=1  AffineConversion=off
  PS-Simulink Converter2 : nesl_utility/PS-Simulink Converter  PhysicalDomain=network_engine_domain  SubClassName=ps_output  LeftPortType=input  RightPortType=output  PseudoPeriodic=off  Frequencies=[]  Unit=1  AffineConversion=off
  Transform Sensor : sm_lib/Frames and Transforms/Transform Sensor  MeasurementFrame=Base  SenseAngle=off  SenseAxis=off  SenseAngle1=off  SenseAngle2=off  SenseAngle3=off  SenseQ=off  SenseR=off  SenseOmegaX=off  SenseOmegaY=off  SenseOmegaZ=off  SenseOmega1=off  SenseOmega2=off  SenseOmega3=off  SenseQDot=off  SenseRDot=off  SenseAlphaX=off  SenseAlphaY=off  SenseAlphaZ=off  SenseAlpha1=off  SenseAlpha2=off  SenseAlpha3=off  SenseQDDot=off  SenseRDDot=off  SenseX=on  SenseY=on  SenseZ=on  SenseRad=off  SenseAzim=off  SenseDist=off  SenseInc=off  SenseXDot=off  SenseYDot=off  SenseZDot=off  SenseRadDot=off  SenseAzimDot=off  SenseDistDot=off  SenseIncDot=off  SenseXDDot=off  SenseYDDot=off  SenseZDDot=off  SenseRadDDot=off  SenseAzimDDot=off  SenseDistDDot=off  SenseIncDDot=off
  F : PMIOPort  Port=1  Side=Left
  B : PMIOPort  Port=2  Side=Left
  x : Outport
  y : Outport  Port=2
  z : Outport  Port=3
  wires:
  PS-Simulink Converter1/1 -> y/1
  PS-Simulink Converter2/1 -> z/1
  PS-Simulink Converter/1 -> x/1
  connections:
  PS-Simulink Converter2/LConn1 -- Transform Sensor/RConn4
  PS-Simulink Converter/LConn1 -- Transform Sensor/RConn2
  PS-Simulink Converter1/LConn1 -- Transform Sensor/RConn3
  B/RConn1 -- Transform Sensor/LConn1
  Transform Sensor/RConn1 -- F/RConn1

== system Flexible_Beam_LP_Modes_GenSS/Wall Conn ==
  note: Variant Subsystem
  Fixed : Subsystem  VariantControl=Fixed
      mask Display: image(imread('Weld_Image.png'))
  Rotate : Subsystem  VariantControl=Rotate
      mask Display: image(imread('Rev_Image.png'))
  B : PMIOPort  Port=1  Side=Left
  F : PMIOPort  Port=2  Side=Right

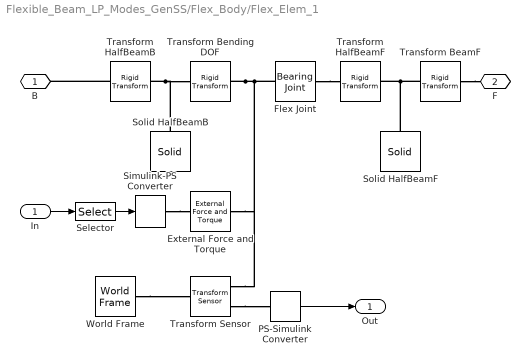
== system Flexible_Beam_LP_Modes_GenSS/Flex_Body/Flex_Elem_1 ==
  In : Inport
  " Transform BeamF" : sm_lib/Frames and Transforms/Rigid Transform  TranslationMethod=StandardAxis  TranslationStandardOffset=length/4  TranslationLengthUnit=m  TranslationStandardAxis=+Z  TranslationCartesianOffset=[0 0 0]  TranslationROffset=0  TranslationROffsetUnits=m  TranslationZOffset=0  TranslationZOffsetUnits=m  TranslationThetaOffset=0  TranslationThetaOffsetUnits=deg  RotationMethod=None  RotationAngleUnits=deg  RotationStandardAxis=+Z  RotationAngle=0  RotationArbitraryAxis=[0 0 1]  FollAlignAxisA=+X  BaseAlignAxisA=+Y  FollAlignAxisB=+Y  BaseAlignAxisB=+Z  RotationSequenceAxes=FollowerAxes  RotationSequence=XYX  RotationSequenceAngles=[0 0 0]  RotationSequenceAnglesUnits=deg  RotationMatrix=[1 0 0; 0 1 0; 0 0 1]
  External Force and Torque : sm_lib/Forces and Torques/External Force and Torque  ForceResolutionFrame=AttachedFrame  EnableForceX=off  EnableForceY=off  EnableForceZ=off  EnableForce=on  TorqueResolutionFrame=AttachedFrame  EnableTorqueX=off  EnableTorqueY=off  EnableTorqueZ=off  EnableTorque=off
  Flex Joint : sm_lib/Joints/Bearing Joint  SenseConstraintForce=off  SenseConstraintForceX=off  SenseConstraintForceY=off  SenseConstraintForceZ=off  SenseConstraintTorque=off  SenseConstraintTorqueX=off  SenseConstraintTorqueY=off  SenseConstraintTorqueZ=off  SenseTotalForce=off  SenseTotalForceX=off  SenseTotalForceY=off  SenseTotalForceZ=off  SenseTotalTorque=off  SenseTotalTorqueX=off  SenseTotalTorqueY=off  SenseTotalTorqueZ=off  CompositeWrenchDir=FollowerOnBase  CompositeWrenchFrame=BaseFrame  PzEquilibriumPosition=0  PzEquilibriumPositionUnits=m  PzSpringStiffness=kelongz  PzSpringStiffnessUnits=N/m  PzDampingCoefficient=b  PzDampingCoefficientUnits=N/(m/s)  PzTorqueActuationMode=NoTorque  PzMotionActuationMode=ComputedMotion  PzSensePosition=off  PzSenseVelocity=off  PzSenseAcceleration=off  PzSenseTorqueForce=off  PzPositionTargetSpecify=off  PzPositionTargetPriority=High  PzPositionTargetValue=0  PzPositionTargetValueUnits=m  PzVelocityTargetSpecify=off  PzVelocityTargetPriority=High  PzVelocityTargetValue=0  PzVelocityTargetValueUnits=m/s  RxEquilibriumPosition=0  RxEquilibriumPositionUnits=deg  RxSpringStiffness=kbendingx  RxSpringStiffnessUnits=N*m/rad  RxDampingCoefficient=b  RxDampingCoefficientUnits=N*m/(rad/s)  RxTorqueActuationMode=NoTorque  RxMotionActuationMode=ComputedMotion  RxSensePosition=off  RxSenseVelocity=off  RxSenseAcceleration=off  RxSenseTorqueForce=off  RxPositionTargetSpecify=off  RxPositionTargetPriority=High  RxPositionTargetValue=0  RxPositionTargetValueUnits=deg  RxVelocityTargetSpecify=off  RxVelocityTargetPriority=High  RxVelocityTargetValue=0  RxVelocityTargetValueUnits=deg/s  RyEquilibriumPosition=0  RyEquilibriumPositionUnits=deg  RySpringStiffness=kbendingy  RySpringStiffnessUnits=N*m/rad  RyDampingCoefficient=b  RyDampingCoefficientUnits=N*m/(rad/s)  RyTorqueActuationMode=NoTorque  RyMotionActuationMode=ComputedMotion  RySensePosition=off  RySenseVelocity=off  RySenseAcceleration=off  RySenseTorqueForce=off  RyPositionTargetSpecify=off  RyPositionTargetPriority=High  RyPositionTargetValue=0  RyPositionTargetValueUnits=deg  RyVelocityTargetSpecify=off  RyVelocityTargetPriority=High  RyVelocityTargetValue=0  RyVelocityTargetValueUnits=deg/s  RzEquilibriumPosition=0  RzEquilibriumPositionUnits=deg  RzSpringStiffness=ktwistz  RzSpringStiffnessUnits=N*m/rad  RzDampingCoefficient=b  RzDampingCoefficientUnits=N*m/(rad/s)  RzTorqueActuationMode=NoTorque  RzMotionActuationMode=ComputedMotion  RzSensePosition=off  RzSenseVelocity=off  RzSenseAcceleration=off  RzSenseTorqueForce=off  RzPositionTargetSpecify=off  RzPositionTargetPriority=High  RzPositionTargetValue=0  RzPositionTargetValueUnits=deg  RzVelocityTargetSpecify=off  RzVelocityTargetPriority=High  RzVelocityTargetValue=0  RzVelocityTargetValueUnits=deg/s
      settings: SourceProductName=Simscape Multibody  SourceProductBaseCode=MS
  PS-Simulink Converter : nesl_utility/PS-Simulink Converter  PhysicalDomain=network_engine_domain  SubClassName=ps_output  LeftPortType=input  RightPortType=output  PseudoPeriodic=off  Frequencies=[]  Unit=1  AffineConversion=off
  Selector : Selector  InputPortWidth=3*numelem  IndexOptions=Index vector (dialog)  Indices=[1 2 3]  OutputSizes=1
  Simulink-PS Converter : nesl_utility/Simulink-PS Converter  PhysicalDomain=network_engine_domain  SubClassName=ps_input  LeftPortType=input  RightPortType=output  PseudoPeriodic=off  Frequencies=[]  NoiseDistribution=none  NoiseParameters=[]  Unit=1  AffineConversion=off  FilteringAndDerivatives=zero  SimscapeFilterOrder=1  InputFilterTimeConstant=0.001  UdotUserProvided=1
  Solid HalfBeamB : sm_lib/Body Elements/Solid  InertiaType=CalculateFromGeometry  Mass=1  MassUnits=kg  CenterOfMass=[0 0 0]  CenterOfMassUnits=m  MomentsOfInertia=[1 1 1]  MomentsOfInertiaUnits=kg*m^2  ProductsOfInertia=[0 0 0]  ProductsOfInertiaUnits=kg*m^2  DensityBased=on  Density=rho  DensityUnits=kg/(m^3)  DoExposeReferenceFrame=on  SerializedFrames=<Frames/>  GraphicType=FromGeometry  MarkerShape=Sphere  MarkerSize=10  MarkerSizeUnits=m  GraphicVisPropType=SimpleVisualProperties  GraphicDiffuseColor=[0.5 0.5 0.5]  GraphicSpecularColor=[0.5 0.5 0.5 1.0]  GraphicAmbientColor=[0.15 0.15 0.15 1.0]  GraphicEmissiveColor=[0.0 0.0 0.0 1.0]  GraphicShininess=75  GraphicOpacity=1.0  GeometryShape=GeneralExtrusion  RectangleSize=[1 1]  RectangleSizeUnits=m  BrickDimensions=[1 1 1]  BrickDimensionUnits=m  CylinderRadius=1  CylinderRadiusUnits=m  CylinderLength=1  CylinderLengthUnits=m  SphereRadius=1  SphereRadiusUnits=m  EllipsoidRadii=[1 1 1]  EllipsoidRadiiUnits=m  ExtrusionCrossSection=extrusion_data  ExtrusionCrossSectionUnits=m  ExtrusionLength=length/2  ExtrusionLengthUnits=m  PolygonNumSides=3  PolygonOuterRadius=1  PolygonOuterRadiusUnits=m  ExtGeomFileType=STL  ExtGeomFileUnits=m  RevolutionCrossSection=[1 1; 1 -1; 2 -1; 2 1]  RevolutionCrossSectionUnits=m  RevolutionExtent=Full  RevolutionAngle=180  RevolutionAngleUnits=deg
  Solid HalfBeamF : sm_lib/Body Elements/Solid  InertiaType=CalculateFromGeometry  Mass=1  MassUnits=kg  CenterOfMass=[0 0 0]  CenterOfMassUnits=m  MomentsOfInertia=[1 1 1]  MomentsOfInertiaUnits=kg*m^2  ProductsOfInertia=[0 0 0]  ProductsOfInertiaUnits=kg*m^2  DensityBased=on  Density=rho  DensityUnits=kg/(m^3)  DoExposeReferenceFrame=on  SerializedFrames=<Frames/>  GraphicType=FromGeometry  MarkerShape=Sphere  MarkerSize=10  MarkerSizeUnits=m  GraphicVisPropType=SimpleVisualProperties  GraphicDiffuseColor=[0.5 0.5 0.5]  GraphicSpecularColor=[0.5 0.5 0.5 1.0]  GraphicAmbientColor=[0.15 0.15 0.15 1.0]  GraphicEmissiveColor=[0.0 0.0 0.0 1.0]  GraphicShininess=75  GraphicOpacity=1.0  GeometryShape=GeneralExtrusion  RectangleSize=[1 1]  RectangleSizeUnits=m  BrickDimensions=[1 1 1]  BrickDimensionUnits=m  CylinderRadius=1  CylinderRadiusUnits=m  CylinderLength=1  CylinderLengthUnits=m  SphereRadius=1  SphereRadiusUnits=m  EllipsoidRadii=[1 1 1]  EllipsoidRadiiUnits=m  ExtrusionCrossSection=extrusion_data  ExtrusionCrossSectionUnits=m  ExtrusionLength=length/2  ExtrusionLengthUnits=m  PolygonNumSides=3  PolygonOuterRadius=1  PolygonOuterRadiusUnits=m  ExtGeomFileType=STL  ExtGeomFileUnits=m  RevolutionCrossSection=[1 1; 1 -1; 2 -1; 2 1]  RevolutionCrossSectionUnits=m  RevolutionExtent=Full  RevolutionAngle=180  RevolutionAngleUnits=deg
  Transform Bending DOF : sm_lib/Frames and Transforms/Rigid Transform  TranslationMethod=StandardAxis  TranslationStandardOffset=length/4  TranslationLengthUnit=m  TranslationStandardAxis=+Z  TranslationCartesianOffset=[0 0 0]  TranslationROffset=0  TranslationROffsetUnits=m  TranslationZOffset=0  TranslationZOffsetUnits=m  TranslationThetaOffset=0  TranslationThetaOffsetUnits=deg  RotationMethod=None  RotationAngleUnits=deg  RotationStandardAxis=+Y  RotationAngle=90  RotationArbitraryAxis=[0 0 1]  FollAlignAxisA=+X  BaseAlignAxisA=+Y  FollAlignAxisB=+Y  BaseAlignAxisB=+Z  RotationSequenceAxes=FollowerAxes  RotationSequence=XYX  RotationSequenceAngles=[0 0 0]  RotationSequenceAnglesUnits=deg  RotationMatrix=[1 0 0; 0 1 0; 0 0 1]
  Transform HalfBeamB : sm_lib/Frames and Transforms/Rigid Transform  TranslationMethod=StandardAxis  TranslationStandardOffset=length/4  TranslationLengthUnit=m  TranslationStandardAxis=+Z  TranslationCartesianOffset=[0 0 0]  TranslationROffset=0  TranslationROffsetUnits=m  TranslationZOffset=0  TranslationZOffsetUnits=m  TranslationThetaOffset=0  TranslationThetaOffsetUnits=deg  RotationMethod=None  RotationAngleUnits=deg  RotationStandardAxis=+Z  RotationAngle=0  RotationArbitraryAxis=[0 0 1]  FollAlignAxisA=+X  BaseAlignAxisA=+Y  FollAlignAxisB=+Y  BaseAlignAxisB=+Z  RotationSequenceAxes=FollowerAxes  RotationSequence=XYX  RotationSequenceAngles=[0 0 0]  RotationSequenceAnglesUnits=deg  RotationMatrix=[1 0 0; 0 1 0; 0 0 1]
  Transform HalfBeamF : sm_lib/Frames and Transforms/Rigid Transform  TranslationMethod=StandardAxis  TranslationStandardOffset=-length/4  TranslationLengthUnit=m  TranslationStandardAxis=+Z  TranslationCartesianOffset=[0 0 0]  TranslationROffset=0  TranslationROffsetUnits=m  TranslationZOffset=0  TranslationZOffsetUnits=m  TranslationThetaOffset=0  TranslationThetaOffsetUnits=deg  RotationMethod=None  RotationAngleUnits=deg  RotationStandardAxis=+Y  RotationAngle=90  RotationArbitraryAxis=[0 0 1]  FollAlignAxisA=+X  BaseAlignAxisA=+Y  FollAlignAxisB=+Y  BaseAlignAxisB=+Z  RotationSequenceAxes=FollowerAxes  RotationSequence=XYX  RotationSequenceAngles=[0 0 0]  RotationSequenceAnglesUnits=deg  RotationMatrix=[1 0 0; 0 1 0; 0 0 1]
  Transform Sensor : sm_lib/Frames and Transforms/Transform Sensor  MeasurementFrame=World  SenseAngle=off  SenseAxis=off  SenseAngle1=off  SenseAngle2=off  SenseAngle3=off  SenseQ=off  SenseR=off  SenseOmegaX=off  SenseOmegaY=off  SenseOmegaZ=on  SenseOmega1=off  SenseOmega2=off  SenseOmega3=off  SenseQDot=off  SenseRDot=off  SenseAlphaX=off  SenseAlphaY=off  SenseAlphaZ=off  SenseAlpha1=off  SenseAlpha2=off  SenseAlpha3=off  SenseQDDot=off  SenseRDDot=off  SenseX=off  SenseY=off  SenseZ=off  SenseRad=off  SenseAzim=off  SenseDist=off  SenseInc=off  SenseXDot=off  SenseYDot=off  SenseZDot=off  SenseRadDot=off  SenseAzimDot=off  SenseDistDot=off  SenseIncDot=off  SenseXDDot=off  SenseYDDot=off  SenseZDDot=off  SenseRadDDot=off  SenseAzimDDot=off  SenseDistDDot=off  SenseIncDDot=off
  World Frame : sm_lib/Frames and Transforms/World Frame
  B : PMIOPort  Port=1  Side=Left
  F : PMIOPort  Port=2  Side=Right
  Out : Outport
  wires:
  PS-Simulink Converter/1 -> Out/1
  Selector/1 -> Simulink-PS Converter/1
  In/1 -> Selector/1
  connections:
  Flex Joint/RConn1 -- Transform HalfBeamF/RConn1
  Transform Sensor/RConn2 -- PS-Simulink Converter/LConn1
  World Frame/RConn1 -- Transform Sensor/LConn1
  Simulink-PS Converter/RConn1 -- External Force and Torque/LConn1
  Transform Bending DOF/RConn1 -- Flex Joint/LConn1 -- External Force and Torque/RConn1 -- Transform Sensor/RConn1
  Transform HalfBeamB/RConn1 -- Transform Bending DOF/LConn1 -- Solid HalfBeamB/RConn1
  Solid HalfBeamF/RConn1 -- " Transform BeamF"/LConn1 -- Transform HalfBeamF/LConn1
  Transform HalfBeamB/LConn1 -- B/RConn1
  " Transform BeamF"/RConn1 -- F/RConn1
